simulink model "Ex7_3"  (Simulink 6.0)
settings: Solver=FixedStepDiscrete  SolverMode=SingleTasking  StartTime=0.0  StopTime=Ts*10  FixedStep=Ts  RelTol=1e-3  AbsTol=1e-6
values from neighbouring files (symbols this model uses):
  Ampl = 10^(Amp_dB/20)    (= 0.312607936712)    [Ex7_3Launch.m]
  delta1 = (A1+1)/(A1+2)    (= 0.99999999)    [Ex7_3Launch.m]
  delta2 = (A2+1)/(A2+2)    (= 0.99999999)    [Ex7_3Launch.m]
  delta3 = (A3+1)/(A3+2)    (= 0.99999999)    [Ex7_3Launch.m]
  delta4 = (A4+1)/(A4+2)    (= 0.99999999)    [Ex7_3Launch.m]
  finrad = Fin*2*pi    (= 66024.9874799)    [Ex7_3Launch.m]
  gain1 = A1/(A1+2)    (= 0.99999998)    [Ex7_3Launch.m]
  gain2 = A2/(A2+2)    (= 0.99999998)    [Ex7_3Launch.m]
  gain3 = A3/(A3+2)    (= 0.99999998)    [Ex7_3Launch.m]
  gain4 = A4/(A4+2)    (= 0.99999998)    [Ex7_3Launch.m]
  sat1 = 1.95    [Ex7_3Launch.m]
  sat2 = 4    [Ex7_3Launch.m]
  sat3 = 4    [Ex7_3Launch.m]
  sat4 = 4    [Ex7_3Launch.m]
  scal1 = 1    [Ex7_3Launch.m]
  scal2 = 1    [Ex7_3Launch.m]
  Ts = 1/Fs    (= 3.54308390023e-07)    [Ex7_3Launch.m]
settings Model: Creator=francomaloberti  LastModifiedBy=Cri  ExtModeAutoUpdateStatusClock=off
settings DataIOCC: LimitDataPoints=off  SignalLoggingName=sigsOut
settings OptimizationCC: BooleanDataType=off  InlineInvariantSignals=off
settings DebuggingCC: SolverPrmCheckMsg=none
settings HardwareCC: TargetUnknown=on

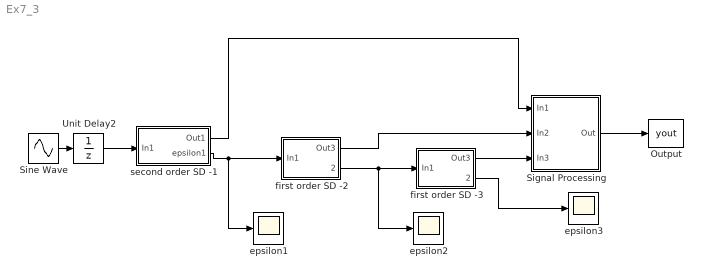
== system Ex7_3 ==
  Output : ToWorkspace  VariableName=yout  SampleTime=-1  SaveFormat=Array
  Signal Processing : Subsystem
      mask Display: color('red');disp('Digital\nSignal\nProcessing')
  Sine Wave : Sin  Amplitude=Ampl  Frequency=finrad  SampleTime=0
  Unit Delay2 : UnitDelay  SampleTime=Ts
  epsilon1 : Scope
      settings: TimeRange=0.003  YMin=-3  YMax=3
  epsilon2 : Scope
      settings: TimeRange=0.003  YMin=-3  YMax=3  SaveName=ScopeData2
  epsilon3 : Scope
      settings: TimeRange=0.003  YMin=-3  YMax=2
  first order SD -2 : Subsystem
      mask Display:
      | plot([20 10 20 10 20 30 40 20], [35 35 25 15 15 35 15 15])
      | port_label('output', 1, 'y');
      | port_label('output', 2, 'err')
  first order SD -3 : Subsystem
      mask Display:
      | plot([20 10 20 10 20 30 40 20], [35 35 25 15 15 35 15 15])
      | port_label('output', 1, 'y');
      | port_label('output', 2, 'err')
  second order SD -1 : Subsystem
      mask Display:
      | plot([20 10 20 10 20 30 40 20], [35 35 25 15 15 35 15 15])
      | port_label('output', 1, 'y');
      | port_label('output', 2, 'err')
  wires:
  Sine Wave/1 -> Unit Delay2/1
  Unit Delay2/1 -> second order SD -1/1(In1)
  second order SD -1/2(epsilon1) -> first order SD -2/1(In1), epsilon1/1
  first order SD -2/2(epsilon2) -> first order SD -3/1(In1), epsilon2/1
  first order SD -3/2(epsilon3) -> epsilon3/1
  first order SD -2/1(Out3) -> Signal Processing/2(In2)
  second order SD -1/1(Out1) -> Signal Processing/1(In1)
  first order SD -3/1(Out3) -> Signal Processing/3(In3)
  Signal Processing/1(Out) -> Output/1

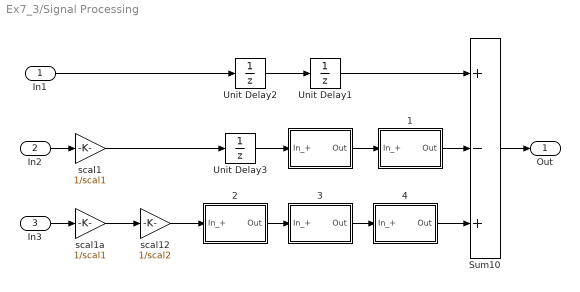
== system Ex7_3/Signal Processing ==
  In1 : Inport  Port=1  LatchInput=off
  In2 : Inport  Port=2  LatchInput=off
  In3 : Inport  Port=3  LatchInput=off
  " " : Subsystem
      mask Display: dpoly([1 -1], 1, 'z-1')
  " 1" : Subsystem
      mask Display: dpoly([1 -1], 1, 'z-1')
  " 2" : Subsystem
      mask Display: dpoly([1 -1], 1, 'z-1')
  " 3" : Subsystem
      mask Display: dpoly([1 -1], 1, 'z-1')
  " 4" : Subsystem
      mask Display: dpoly([1 -1], 1, 'z-1')
  Sum10 : Sum  Inputs=+-+  SaturateOnIntegerOverflow=on  InputSameDT=on
  Unit Delay1 : UnitDelay  SampleTime=Ts
  Unit Delay2 : UnitDelay  SampleTime=Ts
  Unit Delay3 : UnitDelay  SampleTime=Ts
  scal1 : Gain  Gain=1/scal1  SaturateOnIntegerOverflow=on
  scal12 : Gain  Gain=1/scal2  SaturateOnIntegerOverflow=on
  scal1a : Gain  Gain=1/scal1  SaturateOnIntegerOverflow=on
  Out : Outport
  wires:
  In1/1 -> Unit Delay2/1
  Unit Delay2/1 -> Unit Delay1/1
  In2/1 -> scal1/1
  " "/1(Out) -> " 1"/1(In_+)
  Unit Delay3/1 -> " "/1(In_+)
  " 2"/1(Out) -> " 3"/1(In_+)
  In3/1 -> scal1a/1
  " 3"/1(Out) -> " 4"/1(In_+)
  Unit Delay1/1 -> Sum10/1
  " 1"/1(Out) -> Sum10/2
  " 4"/1(Out) -> Sum10/3
  Sum10/1 -> Out/1
  scal1/1 -> Unit Delay3/1
  scal1a/1 -> scal12/1
  scal12/1 -> " 2"/1(In_+)

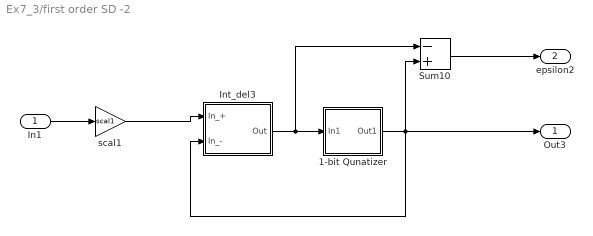
== system Ex7_3/first order SD -2 ==
  In1 : Inport  Port=1  LatchInput=off
  1-bit Qunatizer : Subsystem
      mask Display: plot([25 30 30 35], [0 0 15 15]);
  Int_del3 : Subsystem
      mask Display:
      | patch([10 40 10 10], [0 20 40 0],[1 0 1])
      | plot([10 40 10 10], [0 20 40 0])
      | plot([0 10], [8 8])
      | plot([0 10], [28 28])
      | dpoly([0 1], [1 -1], 'z-')
      | port_label('input', 1, '+')
      | port_label('input', 2, '-')
  Sum10 : Sum  Inputs=-+  SaturateOnIntegerOverflow=on  InputSameDT=on
  scal1 : Gain  Gain=scal1  SaturateOnIntegerOverflow=on
  Out3 : Outport
  epsilon2 : Outport  Port=2
  wires:
  1-bit Qunatizer/1(Out1) -> Sum10/2, Out3/1, Int_del3/2(In_-)
  Int_del3/1(Out) -> 1-bit Qunatizer/1(In1), Sum10/1
  In1/1 -> scal1/1
  Sum10/1 -> epsilon2/1
  scal1/1 -> Int_del3/1(In_+)

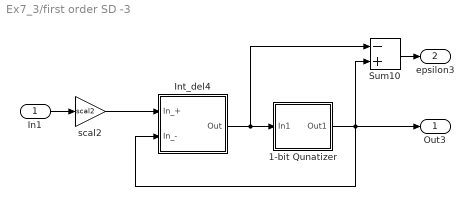
== system Ex7_3/first order SD -3 ==
  In1 : Inport  Port=1  LatchInput=off
  1-bit Qunatizer : Subsystem
      mask Display: plot([25 30 30 35], [0 0 15 15]);
  Int_del4 : Subsystem
      mask Display:
      | patch([10 40 10 10], [0 20 40 0],[1 0 1])
      | plot([10 40 10 10], [0 20 40 0])
      | plot([0 10], [8 8])
      | plot([0 10], [28 28])
      | dpoly([0 1], [1 -1], 'z-')
      | port_label('input', 1, '+')
      | port_label('input', 2, '-')
  Sum10 : Sum  Inputs=-+  SaturateOnIntegerOverflow=on  InputSameDT=on
  scal2 : Gain  Gain=scal2  SaturateOnIntegerOverflow=on
  Out3 : Outport
  epsilon3 : Outport  Port=2
  wires:
  In1/1 -> scal2/1
  Int_del4/1(Out) -> 1-bit Qunatizer/1(In1), Sum10/1
  1-bit Qunatizer/1(Out1) -> Out3/1, Sum10/2, Int_del4/2(In_-)
  Sum10/1 -> epsilon3/1
  scal2/1 -> Int_del4/1(In_+)

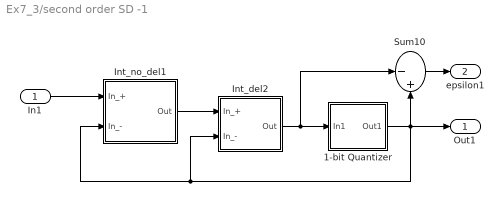
== system Ex7_3/second order SD -1 ==
  In1 : Inport  Port=1  LatchInput=off
  1-bit Quantizer : Subsystem
      mask Display: plot([25 30 30 35], [0 0 15 15]);
  Int_del2 : Subsystem
      mask Display:
      | patch([10 40 10 10], [0 20 40 0],[1 0 1])
      | plot([10 40 10 10], [0 20 40 0])
      | plot([0 10], [8 8])
      | plot([0 10], [28 28])
      | dpoly([0 1], [1 -1], 'z-')
      | port_label('input', 1, '+')
      | port_label('input', 2, '-')
  Int_no_del1 : Subsystem
      mask Display:
      | patch([10 40 10 10], [0 20 40 0],[0 1 1])
      | plot([10 40 10 10], [0 20 40 0])
      | plot([0 10], [8 8])
      | plot([0 10], [28 28])
      | dpoly([1], [1 -1], 'z-')
      | port_label('input', 1, '+')
      | port_label('input', 2, '-')
  Sum10 : Sum  Inputs=|-+  SaturateOnIntegerOverflow=on  InputSameDT=on
  Out1 : Outport
  epsilon1 : Outport  Port=2
  wires:
  In1/1 -> Int_no_del1/1(In_+)
  Int_no_del1/1(Out) -> Int_del2/1(In_+)
  Int_del2/1(Out) -> 1-bit Quantizer/1(In1), Sum10/1
  1-bit Quantizer/1(Out1) -> Out1/1, Sum10/2, Int_no_del1/2(In_-), Int_del2/2(In_-)
  Sum10/1 -> epsilon1/1

== system Ex7_3/Signal Processing/  ==
  In_+ : Inport  Port=1  LatchInput=off
  Sum10 : Sum  Inputs=+-  SaturateOnIntegerOverflow=on  InputSameDT=on
  Unit Delay1 : UnitDelay  SampleTime=Ts
  Out : Outport
  wires:
  In_+/1 -> Unit Delay1/1, Sum10/1
  Unit Delay1/1 -> Sum10/2
  Sum10/1 -> Out/1

== system Ex7_3/Signal Processing/ 1 ==
  In_+ : Inport  Port=1  LatchInput=off
  Sum10 : Sum  Inputs=+-  SaturateOnIntegerOverflow=on  InputSameDT=on
  Unit Delay1 : UnitDelay  SampleTime=Ts
  Out : Outport
  wires:
  In_+/1 -> Unit Delay1/1, Sum10/1
  Unit Delay1/1 -> Sum10/2
  Sum10/1 -> Out/1

== system Ex7_3/Signal Processing/ 2 ==
  In_+ : Inport  Port=1  LatchInput=off
  Sum10 : Sum  Inputs=+-  SaturateOnIntegerOverflow=on  InputSameDT=on
  Unit Delay1 : UnitDelay  SampleTime=Ts
  Out : Outport
  wires:
  In_+/1 -> Unit Delay1/1, Sum10/1
  Unit Delay1/1 -> Sum10/2
  Sum10/1 -> Out/1

== system Ex7_3/Signal Processing/ 3 ==
  In_+ : Inport  Port=1  LatchInput=off
  Sum10 : Sum  Inputs=+-  SaturateOnIntegerOverflow=on  InputSameDT=on
  Unit Delay1 : UnitDelay  SampleTime=Ts
  Out : Outport
  wires:
  In_+/1 -> Unit Delay1/1, Sum10/1
  Unit Delay1/1 -> Sum10/2
  Sum10/1 -> Out/1

== system Ex7_3/Signal Processing/ 4 ==
  In_+ : Inport  Port=1  LatchInput=off
  Sum10 : Sum  Inputs=+-  SaturateOnIntegerOverflow=on  InputSameDT=on
  Unit Delay1 : UnitDelay  SampleTime=Ts
  Out : Outport
  wires:
  In_+/1 -> Unit Delay1/1, Sum10/1
  Unit Delay1/1 -> Sum10/2
  Sum10/1 -> Out/1

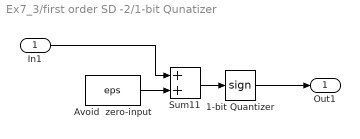
== system Ex7_3/first order SD -2/1-bit Qunatizer ==
  In1 : Inport  Port=1  LatchInput=off
  1-bit Quantizer : Signum
  Avoid  zero-input : Constant  Value=eps
  Sum11 : Sum  SaturateOnIntegerOverflow=on  InputSameDT=on
  Out1 : Outport
  wires:
  Avoid  zero-input/1 -> Sum11/2
  Sum11/1 -> 1-bit Quantizer/1
  In1/1 -> Sum11/1
  1-bit Quantizer/1 -> Out1/1

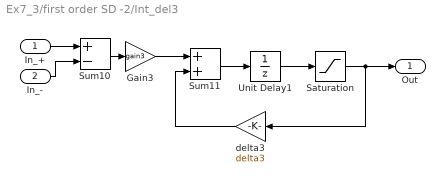
== system Ex7_3/first order SD -2/Int_del3 ==
  In_+ : Inport  Port=1  LatchInput=off
  In_- : Inport  Port=2  LatchInput=off
  Gain3 : Gain  Gain=gain3  SaturateOnIntegerOverflow=on
  Saturation : Saturate  UpperLimit=sat3  LowerLimit=-sat3
  Sum10 : Sum  Inputs=+-  SaturateOnIntegerOverflow=on  InputSameDT=on
  Sum11 : Sum  SaturateOnIntegerOverflow=on  InputSameDT=on
  Unit Delay1 : UnitDelay  SampleTime=Ts
  delta3 : Gain  Orientation=left  Gain=delta3  SaturateOnIntegerOverflow=on
  Out : Outport
  wires:
  delta3/1 -> Sum11/2
  Gain3/1 -> Sum11/1
  Sum10/1 -> Gain3/1
  Sum11/1 -> Unit Delay1/1
  In_-/1 -> Sum10/2
  In_+/1 -> Sum10/1
  Unit Delay1/1 -> Saturation/1
  Saturation/1 -> delta3/1, Out/1

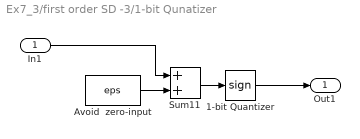
== system Ex7_3/first order SD -3/1-bit Qunatizer ==
  In1 : Inport  Port=1  LatchInput=off
  1-bit Quantizer : Signum
  Avoid  zero-input : Constant  Value=eps
  Sum11 : Sum  SaturateOnIntegerOverflow=on  InputSameDT=on
  Out1 : Outport
  wires:
  1-bit Quantizer/1 -> Out1/1
  In1/1 -> Sum11/1
  Sum11/1 -> 1-bit Quantizer/1
  Avoid  zero-input/1 -> Sum11/2

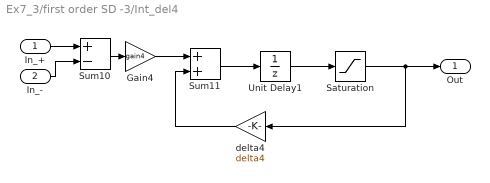
== system Ex7_3/first order SD -3/Int_del4 ==
  In_+ : Inport  Port=1  LatchInput=off
  In_- : Inport  Port=2  LatchInput=off
  Gain4 : Gain  Gain=gain4  SaturateOnIntegerOverflow=on
  Saturation : Saturate  UpperLimit=sat4  LowerLimit=-sat4
  Sum10 : Sum  Inputs=+-  SaturateOnIntegerOverflow=on  InputSameDT=on
  Sum11 : Sum  SaturateOnIntegerOverflow=on  InputSameDT=on
  Unit Delay1 : UnitDelay  SampleTime=Ts
  delta4 : Gain  Orientation=left  Gain=delta4  SaturateOnIntegerOverflow=on
  Out : Outport
  wires:
  Unit Delay1/1 -> Saturation/1
  In_+/1 -> Sum10/1
  In_-/1 -> Sum10/2
  Sum11/1 -> Unit Delay1/1
  Sum10/1 -> Gain4/1
  Gain4/1 -> Sum11/1
  delta4/1 -> Sum11/2
  Saturation/1 -> Out/1, delta4/1

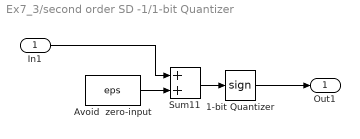
== system Ex7_3/second order SD -1/1-bit Quantizer ==
  In1 : Inport  Port=1  LatchInput=off
  1-bit Quantizer : Signum
  Avoid  zero-input : Constant  Value=eps
  Sum11 : Sum  SaturateOnIntegerOverflow=on  InputSameDT=on
  Out1 : Outport
  wires:
  1-bit Quantizer/1 -> Out1/1
  In1/1 -> Sum11/1
  Sum11/1 -> 1-bit Quantizer/1
  Avoid  zero-input/1 -> Sum11/2

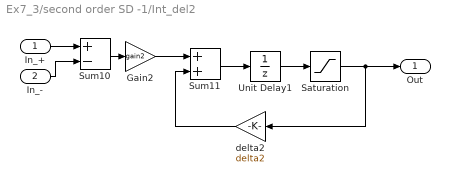
== system Ex7_3/second order SD -1/Int_del2 ==
  In_+ : Inport  Port=1  LatchInput=off
  In_- : Inport  Port=2  LatchInput=off
  Gain2 : Gain  Gain=gain2  SaturateOnIntegerOverflow=on
  Saturation : Saturate  UpperLimit=sat2  LowerLimit=-sat2
  Sum10 : Sum  Inputs=+-  SaturateOnIntegerOverflow=on  InputSameDT=on
  Sum11 : Sum  SaturateOnIntegerOverflow=on  InputSameDT=on
  Unit Delay1 : UnitDelay  SampleTime=Ts
  delta2 : Gain  Orientation=left  Gain=delta2  SaturateOnIntegerOverflow=on
  Out : Outport
  wires:
  Unit Delay1/1 -> Saturation/1
  In_+/1 -> Sum10/1
  In_-/1 -> Sum10/2
  Sum11/1 -> Unit Delay1/1
  Sum10/1 -> Gain2/1
  Gain2/1 -> Sum11/1
  delta2/1 -> Sum11/2
  Saturation/1 -> Out/1, delta2/1

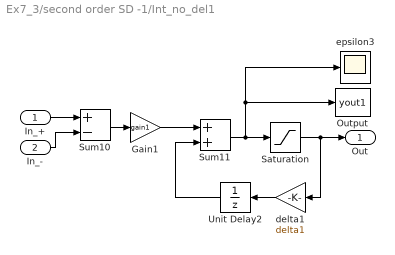
== system Ex7_3/second order SD -1/Int_no_del1 ==
  In_+ : Inport  Port=1  LatchInput=off
  In_- : Inport  Port=2  LatchInput=off
  Gain1 : Gain  Gain=gain1  SaturateOnIntegerOverflow=on
  Output : ToWorkspace  VariableName=yout1  SampleTime=-1  SaveFormat=Array
  Saturation : Saturate  UpperLimit=sat1  LowerLimit=-sat1
  Sum10 : Sum  Inputs=+-  SaturateOnIntegerOverflow=on  InputSameDT=on
  Sum11 : Sum  SaturateOnIntegerOverflow=on  InputSameDT=on
  Unit Delay2 : UnitDelay  Orientation=left  SampleTime=Ts
  delta1 : Gain  Orientation=left  Gain=delta1  SaturateOnIntegerOverflow=on
  epsilon3 : Scope
      settings: TimeRange=0.003  YMin=-3  YMax=2  SaveName=ScopeData3
  Out : Outport
  wires:
  Gain1/1 -> Sum11/1
  Sum10/1 -> Gain1/1
  Sum11/1 -> Saturation/1, epsilon3/1, Output/1
  In_-/1 -> Sum10/2
  In_+/1 -> Sum10/1
  Unit Delay2/1 -> Sum11/2
  delta1/1 -> Unit Delay2/1
  Saturation/1 -> Out/1, delta1/1
